simulink model "iff_sim"  (R2019b)
settings: Solver=VariableStepAuto  StartTime=0.0  StopTime=T  FixedStep=0.001  MaxStep=0.01  RelTol=1e-3
values from neighbouring files (symbols this model uses):
  bsc = 17    [model.mat]
  d_r = [0.01 0.01 0.01 0.01 0.01 0.01]    [model.mat]
  Fi_b_z = in_rlb(12,1)    [fcn_s_rlb.m]    (also in fcn_s_rub.m = in_rub(12,1); model.mat = [0 2.09439510239 4.18879020479 1.0471975512 3.14159265359 5.)
  ka = 11860000    [model.mat]
  ksc = 179000    [model.mat]
  l_r = in_rlb(3,1)    [fcn_s_rlb.m]    (also in fcn_s_rub.m = in_rub(3,1); model.mat = [0.36 0.36 0.36 0.36 0.36 0.36])
  la00 = 0.061    [model.mat]
  linderiv = 0    [model.mat]
  O_lb = in_rlb(4:9,1)    [fcn_s_rlb.m]    (also in model.mat = [0 0 0 0 0 0])
  s_0 = s_d(:,:,1)    [iff_run.m]
  t_dist = 0.1    [model.mat]
  ts_noise = 0.00016    [model.mat]
  v_0 = v_d(:,:,1)    [iff_run.m]
  w_lb = in_rlb(11,1)    [fcn_s_rlb.m]    (also in model.mat = 0.195)
  W_lb = 0.205    [model.mat]
  w_ub = in_rub(11,1)    [fcn_s_rub.m]    (also in model.mat = 0.195)
  W_ub = 0.205    [model.mat]
undefined symbols (not defined in the file or in its folder): Kd, Kdiag, Ki, Kp, q_d, qt_d, qtt_d, t_d, X, Y, Z
libraries: nesl_utility x282, sm_lib x208, dspindex x30, simulink_extras x24, simulink x14, powerlib_meascontrol x1
(part 5 of 14)

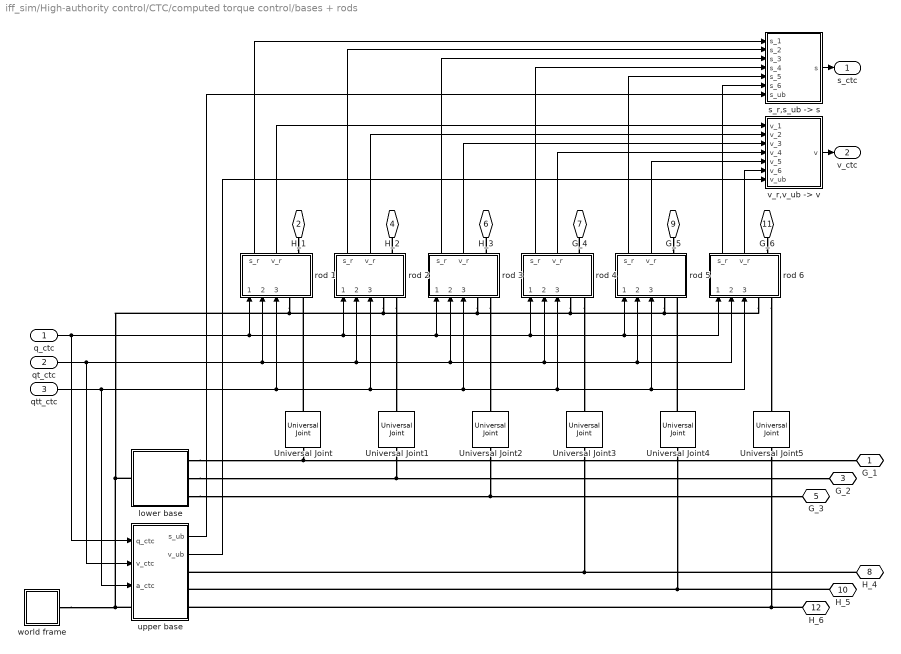
== system iff_sim/High-authority control/CTC/computed torque control/bases + rods ==
  q_ctc : Inport
  qt_ctc : Inport  Port=2
  qtt_ctc : Inport  Port=3
  Universal Joint{,1..5} (6 alike) : sm_lib/Joints/Universal Joint  JointMode=Normal  SenseConstraintForce=off  SenseConstraintForceX=off  SenseConstraintForceY=off  SenseConstraintForceZ=off  SenseConstraintTorque=off  SenseConstraintTorqueX=off  SenseConstraintTorqueY=off  SenseConstraintTorqueZ=off  SenseTotalForce=off  SenseTotalForceX=off  SenseTotalForceY=off  SenseTotalForceZ=off  SenseTotalTorque=off  SenseTotalTorqueX=off  SenseTotalTorqueY=off  SenseTotalTorqueZ=off  CompositeWrenchDir=FollowerOnBase  CompositeWrenchFrame=BaseFrame  RxEquilibriumPosition=0  RxEquilibriumPositionUnits=deg  RxSpringStiffness=0  RxSpringStiffnessUnits=N*m/deg  RxDampingCoefficient=0  RxDampingCoefficientUnits=N*m/(deg/s)  RxTorqueActuationMode=NoTorque  RxMotionActuationMode=ComputedMotion  RxSensePosition=off  RxSenseVelocity=off  RxSenseAcceleration=off  RxSenseTorqueForce=off  RxSenseLowerLimitTorqueForce=off  RxSenseUpperLimitTorqueForce=off  RxLowerLimitSpecify=off  RxLowerLimitBound=-90  RxLowerLimitBoundUnits=deg  RxLowerLimitStiffness=1e4  RxLowerLimitStiffnessUnits=N*m/deg  RxLowerLimitDamping=10  RxLowerLimitDampingUnits=N*m/(deg/s)  RxLowerLimitTransitionRegionWidth=0.1  RxLowerLimitTransitionRegionWidthUnits=deg  RxUpperLimitSpecify=off  RxUpperLimitBound=90  RxUpperLimitBoundUnits=deg  RxUpperLimitStiffness=1e4  RxUpperLimitStiffnessUnits=N*m/deg  RxUpperLimitDamping=10  RxUpperLimitDampingUnits=N*m/(deg/s)  RxUpperLimitTransitionRegionWidth=0.1  RxUpperLimitTransitionRegionWidthUnits=deg  RxPositionTargetSpecify=off  RxPositionTargetPriority=High  RxPositionTargetValue=0  RxPositionTargetValueUnits=deg  RxVelocityTargetSpecify=off  RxVelocityTargetPriority=High  RxVelocityTargetValue=0  RxVelocityTargetValueUnits=deg/s  RyEquilibriumPosition=0  RyEquilibriumPositionUnits=deg  RySpringStiffness=0  RySpringStiffnessUnits=N*m/deg  RyDampingCoefficient=0  RyDampingCoefficientUnits=N*m/(deg/s)  RyTorqueActuationMode=NoTorque  RyMotionActuationMode=ComputedMotion  RySensePosition=off  RySenseVelocity=off  RySenseAcceleration=off  RySenseTorqueForce=off  RySenseLowerLimitTorqueForce=off  RySenseUpperLimitTorqueForce=off  RyLowerLimitSpecify=off  RyLowerLimitBound=-90  RyLowerLimitBoundUnits=deg  RyLowerLimitStiffness=1e4  RyLowerLimitStiffnessUnits=N*m/deg  RyLowerLimitDamping=10  RyLowerLimitDampingUnits=N*m/(deg/s)  RyLowerLimitTransitionRegionWidth=0.1  RyLowerLimitTransitionRegionWidthUnits=deg  RyUpperLimitSpecify=off  RyUpperLimitBound=90  RyUpperLimitBoundUnits=deg  RyUpperLimitStiffness=1e4  RyUpperLimitStiffnessUnits=N*m/deg  RyUpperLimitDamping=10  RyUpperLimitDampingUnits=N*m/(deg/s)  RyUpperLimitTransitionRegionWidth=0.1  RyUpperLimitTransitionRegionWidthUnits=deg  RyPositionTargetSpecify=off  RyPositionTargetPriority=High  RyPositionTargetValue=0  RyPositionTargetValueUnits=deg  RyVelocityTargetSpecify=off  RyVelocityTargetPriority=High  RyVelocityTargetValue=0  RyVelocityTargetValueUnits=deg/s
      settings: SourceProductName=Simscape Multibody
  lower base : Subsystem
  rod 1 : Subsystem  mask{r=1}
  rod 2 : Subsystem  mask{r=2}
  rod 3 : Subsystem  mask{r=3}
  rod 4 : Subsystem  mask{r=4}
  rod 5 : Subsystem  mask{r=5}
  rod 6 : Subsystem  mask{r=6}
  "s_r,s_ub -> s" : MATLAB Function  TreatAsAtomicUnit=on
  upper base : Subsystem
  "v_r,v_ub -> v" : MATLAB Function  TreatAsAtomicUnit=on
  world frame : Subsystem
  G_1 : PMIOPort  Side=Right
  H_1 : PMIOPort  Port=2  Side=Right
  G_2 : PMIOPort  Port=3  Side=Right
  H_2 : PMIOPort  Port=4  Side=Right
  G_3 : PMIOPort  Port=5  Side=Right
  H_3 : PMIOPort  Port=6  Side=Right
  G_4 : PMIOPort  Port=7  Side=Right
  H_4 : PMIOPort  Port=8  Side=Right
  G_5 : PMIOPort  Port=9  Side=Right
  H_5 : PMIOPort  Port=10  Side=Right
  G_6 : PMIOPort  Port=11  Side=Right
  H_6 : PMIOPort  Port=12  Side=Right
  s_ctc : Outport
  v_ctc : Outport  Port=2
  wires:
  q_ctc/1 -> upper base/1(q_ctc), rod 2/1(q_ctc), rod 3/1(q_ctc), rod 4/1(q_ctc), rod 6/1(q_ctc), rod 5/1(q_ctc), rod 1/1(q_ctc)
  qt_ctc/1 -> upper base/2(v_ctc), rod 2/2(v_ctc), rod 3/2(v_ctc), rod 4/2(v_ctc), rod 6/2(v_ctc), rod 5/2(v_ctc), rod 1/2(v_ctc)
  qtt_ctc/1 -> upper base/3(a_ctc), rod 2/3(a_ctc), rod 3/3(a_ctc), rod 4/3(a_ctc), rod 6/3(a_ctc), rod 5/3(a_ctc), rod 1/3(a_ctc)
  rod 4/1(s_r) -> "s_r,s_ub -> s"/4(s_4)
  rod 3/1(s_r) -> "s_r,s_ub -> s"/3(s_3)
  rod 2/1(s_r) -> "s_r,s_ub -> s"/2(s_2)
  rod 1/1(s_r) -> "s_r,s_ub -> s"/1(s_1)
  "s_r,s_ub -> s"/1(s) -> s_ctc/1
  upper base/1(s_ub) -> "s_r,s_ub -> s"/7(s_ub)
  "v_r,v_ub -> v"/1(v) -> v_ctc/1
  rod 4/2(v_r) -> "v_r,v_ub -> v"/4(v_4)
  rod 3/2(v_r) -> "v_r,v_ub -> v"/3(v_3)
  rod 2/2(v_r) -> "v_r,v_ub -> v"/2(v_2)
  rod 1/2(v_r) -> "v_r,v_ub -> v"/1(v_1)
  upper base/2(v_ub) -> "v_r,v_ub -> v"/7(v_ub)
  rod 5/1(s_r) -> "s_r,s_ub -> s"/5(s_5)
  rod 6/1(s_r) -> "s_r,s_ub -> s"/6(s_6)
  rod 5/2(v_r) -> "v_r,v_ub -> v"/5(v_5)
  rod 6/2(v_r) -> "v_r,v_ub -> v"/6(v_6)
  connections:
  lower base/RConn1 -- Universal Joint/LConn1 -- G_1/RConn1
  lower base/RConn2 -- G_2/RConn1 -- Universal Joint1/LConn1
  lower base/RConn3 -- G_3/RConn1 -- Universal Joint2/LConn1
  Universal Joint3/LConn1 -- H_4/RConn1 -- upper base/RConn1
  Universal Joint4/LConn1 -- H_5/RConn1 -- upper base/RConn2
  H_6/RConn1 -- Universal Joint5/LConn1 -- upper base/RConn3
  H_1/RConn1 -- rod 1/RConn1
  Universal Joint/RConn1 -- rod 1/LConn2
  rod 2/LConn2 -- Universal Joint1/RConn1
  rod 2/RConn1 -- H_2/RConn1
  rod 3/RConn1 -- H_3/RConn1
  world frame/RConn1 -- upper base/LConn1 -- lower base/LConn1 -- rod 1/LConn1 -- rod 2/LConn1 -- rod 3/LConn1 -- rod 4/LConn1 -- rod 6/LConn1 -- rod 5/LConn1
  rod 3/LConn2 -- Universal Joint2/RConn1
  rod 4/LConn2 -- Universal Joint3/RConn1
  rod 4/RConn1 -- G_4/RConn1
  Universal Joint4/RConn1 -- rod 5/LConn2
  G_5/RConn1 -- rod 5/RConn1
  G_6/RConn1 -- rod 6/RConn1
  rod 6/LConn2 -- Universal Joint5/RConn1

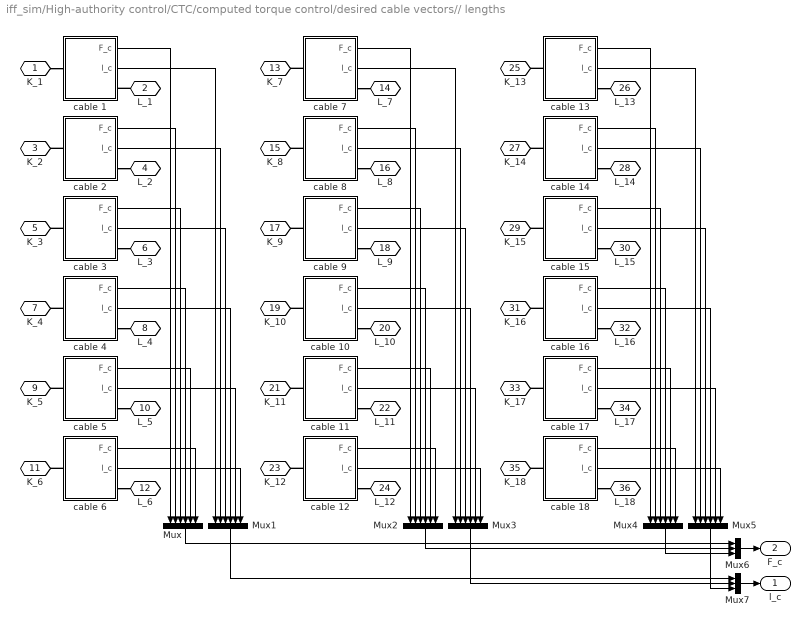
== system iff_sim/High-authority control/CTC/computed torque control/desired cable vectors// lengths ==
  Mux{,1..5} (6 alike) : Mux  Inputs=6
  Mux6 : Mux  Inputs=3
  Mux7 : Mux  Inputs=3
  cable 1 : Subsystem
  cable 10 : Subsystem
  cable 11 : Subsystem
  cable 12 : Subsystem
  cable 13 : Subsystem
  cable 14 : Subsystem
  cable 15 : Subsystem
  cable 16 : Subsystem
  cable 17 : Subsystem
  cable 18 : Subsystem
  cable 2 : Subsystem
  cable 3 : Subsystem
  cable 4 : Subsystem
  cable 5 : Subsystem
  cable 6 : Subsystem
  cable 7 : Subsystem
  cable 8 : Subsystem
  cable 9 : Subsystem
  K_1 : PMIOPort  Side=Left
  L_1 : PMIOPort  Port=2  Side=Left
  K_2 : PMIOPort  Port=3  Side=Left
  L_2 : PMIOPort  Port=4  Side=Left
  K_3 : PMIOPort  Port=5  Side=Left
  L_3 : PMIOPort  Port=6  Side=Left
  K_4 : PMIOPort  Port=7  Side=Left
  L_4 : PMIOPort  Port=8  Side=Left
  K_5 : PMIOPort  Port=9  Side=Left
  L_5 : PMIOPort  Port=10  Side=Left
  K_6 : PMIOPort  Port=11  Side=Left
  L_6 : PMIOPort  Port=12  Side=Left
  K_7 : PMIOPort  Port=13  Side=Left
  L_7 : PMIOPort  Port=14  Side=Left
  K_8 : PMIOPort  Port=15  Side=Left
  L_8 : PMIOPort  Port=16  Side=Left
  K_9 : PMIOPort  Port=17  Side=Left
  L_9 : PMIOPort  Port=18  Side=Left
  K_10 : PMIOPort  Port=19  Side=Left
  L_10 : PMIOPort  Port=20  Side=Left
  K_11 : PMIOPort  Port=21  Side=Left
  L_11 : PMIOPort  Port=22  Side=Left
  K_12 : PMIOPort  Port=23  Side=Left
  L_12 : PMIOPort  Port=24  Side=Left
  K_13 : PMIOPort  Port=25  Side=Left
  L_13 : PMIOPort  Port=26  Side=Left
  K_14 : PMIOPort  Port=27  Side=Left
  L_14 : PMIOPort  Port=28  Side=Left
  K_15 : PMIOPort  Port=29  Side=Left
  L_15 : PMIOPort  Port=30  Side=Left
  K_16 : PMIOPort  Port=31  Side=Left
  L_16 : PMIOPort  Port=32  Side=Left
  K_17 : PMIOPort  Port=33  Side=Left
  L_17 : PMIOPort  Port=34  Side=Left
  K_18 : PMIOPort  Port=35  Side=Left
  L_18 : PMIOPort  Port=36  Side=Left
  l_c : Outport
  F_c : Outport  Port=2
  wires:
  cable 1/1(F_c) -> Mux/1
  cable 2/1(F_c) -> Mux/2
  cable 3/1(F_c) -> Mux/3
  cable 4/1(F_c) -> Mux/4
  cable 5/1(F_c) -> Mux/5
  cable 6/1(F_c) -> Mux/6
  cable 1/2(l_c) -> Mux1/1
  cable 2/2(l_c) -> Mux1/2
  cable 3/2(l_c) -> Mux1/3
  cable 4/2(l_c) -> Mux1/4
  cable 5/2(l_c) -> Mux1/5
  cable 6/2(l_c) -> Mux1/6
  cable 8/2(l_c) -> Mux3/2
  cable 9/1(F_c) -> Mux2/3
  cable 11/1(F_c) -> Mux2/5
  cable 10/2(l_c) -> Mux3/4
  cable 12/2(l_c) -> Mux3/6
  cable 12/1(F_c) -> Mux2/6
  cable 9/2(l_c) -> Mux3/3
  cable 11/2(l_c) -> Mux3/5
  cable 10/1(F_c) -> Mux2/4
  cable 7/1(F_c) -> Mux2/1
  cable 7/2(l_c) -> Mux3/1
  cable 8/1(F_c) -> Mux2/2
  cable 14/2(l_c) -> Mux5/2
  cable 15/1(F_c) -> Mux4/3
  cable 17/1(F_c) -> Mux4/5
  cable 16/2(l_c) -> Mux5/4
  cable 18/2(l_c) -> Mux5/6
  cable 18/1(F_c) -> Mux4/6
  cable 15/2(l_c) -> Mux5/3
  cable 17/2(l_c) -> Mux5/5
  cable 16/1(F_c) -> Mux4/4
  cable 13/1(F_c) -> Mux4/1
  cable 13/2(l_c) -> Mux5/1
  cable 14/1(F_c) -> Mux4/2
  Mux6/1 -> F_c/1
  Mux/1 -> Mux6/1
  Mux2/1 -> Mux6/2
  Mux4/1 -> Mux6/3
  Mux7/1 -> l_c/1
  Mux1/1 -> Mux7/1
  Mux3/1 -> Mux7/2
  Mux5/1 -> Mux7/3
  connections:
  K_1/RConn1 -- cable 1/LConn1
  L_1/RConn1 -- cable 1/RConn1
  cable 2/RConn1 -- L_2/RConn1
  cable 2/LConn1 -- K_2/RConn1
  cable 3/LConn1 -- K_3/RConn1
  cable 3/RConn1 -- L_3/RConn1
  cable 6/RConn1 -- L_6/RConn1
  cable 4/LConn1 -- K_4/RConn1
  cable 5/RConn1 -- L_5/RConn1
  cable 4/RConn1 -- L_4/RConn1
  cable 6/LConn1 -- K_6/RConn1
  cable 5/LConn1 -- K_5/RConn1
  cable 12/RConn1 -- L_12/RConn1
  cable 11/RConn1 -- L_11/RConn1
  cable 7/LConn1 -- K_7/RConn1
  cable 7/RConn1 -- L_7/RConn1
  cable 12/LConn1 -- K_12/RConn1
  cable 8/LConn1 -- K_8/RConn1
  cable 9/RConn1 -- L_9/RConn1
  cable 10/RConn1 -- L_10/RConn1
  cable 10/LConn1 -- K_10/RConn1
  cable 8/RConn1 -- L_8/RConn1
  cable 9/LConn1 -- K_9/RConn1
  cable 11/LConn1 -- K_11/RConn1
  cable 18/RConn1 -- L_18/RConn1
  cable 17/RConn1 -- L_17/RConn1
  cable 13/LConn1 -- K_13/RConn1
  cable 18/LConn1 -- K_18/RConn1
  cable 13/RConn1 -- L_13/RConn1
  cable 16/RConn1 -- L_16/RConn1
  cable 14/LConn1 -- K_14/RConn1
  cable 14/RConn1 -- L_14/RConn1
  cable 16/LConn1 -- K_16/RConn1
  cable 17/LConn1 -- K_17/RConn1
  cable 15/RConn1 -- L_15/RConn1
  cable 15/LConn1 -- K_15/RConn1

== system iff_sim/High-authority control/CTC/computed torque control/q_d,q -> a_ctc ==
  q_d : Inport
  qt_d : Inport  Port=2
  qtt_d : Inport  Port=3
  q : Inport  Port=4
  qt : Inport  Port=5
  Gain : Gain  Gain=Kp
  Gain1 : Gain  Gain=Kd
  Gain2 : Gain  Gain=Ki
  Integrator : Integrator
  Sum : Sum  Inputs=+-|
  Sum1 : Sum  Inputs=+-|
  Sum2 : Sum  Inputs=++++
  To Workspace : ToWorkspace  VariableName=e  SampleTime=-1
  q_ctc : Outport
  qt_ctc : Outport  Port=2
  qtt_ctc : Outport  Port=3
  wires:
  q_d/1 -> Sum/1, q_ctc/1
  qt_d/1 -> Sum1/1, qt_ctc/1
  q/1 -> Sum/2
  qt/1 -> Sum1/2
  Sum2/1 -> qtt_ctc/1
  qtt_d/1 -> Sum2/1
  Sum/1 -> Integrator/1, Gain/1, To Workspace/1
  Gain/1 -> Sum2/2
  Sum1/1 -> Gain1/1
  Gain1/1 -> Sum2/3
  Gain2/1 -> Sum2/4
  Integrator/1 -> Gain2/1

== system iff_sim/High-authority control/CTC/computed torque control/scope q_ctc ==
  in : Inport
  Multiport Selector : dspindex/Multiport Selector  rowsOrCols=Rows  idxCellArray={ 1,2,3,4,5,6}  idxErrMode=Clip Index
  Multiport Selector1 : dspindex/Multiport Selector  rowsOrCols=Rows  idxCellArray={ 7,8,9,10,11,12}  idxErrMode=Clip Index
  Multiport Selector2 : dspindex/Multiport Selector  rowsOrCols=Rows  idxCellArray={ 13,14,15,16,17,18}  idxErrMode=Clip Index
  r = 1-3 : Scope  NumInputPorts=6
  r = 4-6 : Scope  NumInputPorts=6
  ub : Scope  NumInputPorts=6
  wires:
  Multiport Selector/1 -> r = 1-3/1
  Multiport Selector2/2 -> ub/2
  in/1 -> Multiport Selector2/1, Multiport Selector/1, Multiport Selector1/1
  Multiport Selector/2 -> r = 1-3/2
  Multiport Selector1/5 -> r = 4-6/5
  Multiport Selector2/4 -> ub/4
  Multiport Selector/5 -> r = 1-3/5
  Multiport Selector/6 -> r = 1-3/6
  Multiport Selector2/1 -> ub/1
  Multiport Selector/3 -> r = 1-3/3
  Multiport Selector2/5 -> ub/5
  Multiport Selector/4 -> r = 1-3/4
  Multiport Selector1/6 -> r = 4-6/6
  Multiport Selector1/2 -> r = 4-6/2
  Multiport Selector1/4 -> r = 4-6/4
  Multiport Selector1/3 -> r = 4-6/3
  Multiport Selector1/1 -> r = 4-6/1
  Multiport Selector2/3 -> ub/3
  Multiport Selector2/6 -> ub/6

== system iff_sim/High-authority control/CTC/computed torque control/scope qt_ctc ==
  in : Inport
  Multiport Selector : dspindex/Multiport Selector  rowsOrCols=Rows  idxCellArray={ 1,2,3,4,5,6}  idxErrMode=Clip Index
  Multiport Selector1 : dspindex/Multiport Selector  rowsOrCols=Rows  idxCellArray={ 7,8,9,10,11,12}  idxErrMode=Clip Index
  Multiport Selector2 : dspindex/Multiport Selector  rowsOrCols=Rows  idxCellArray={ 13,14,15,16,17,18}  idxErrMode=Clip Index
  r = 1-3 : Scope  NumInputPorts=6
  r = 4-6 : Scope  NumInputPorts=6
  ub : Scope  NumInputPorts=6
  wires:
  Multiport Selector/1 -> r = 1-3/1
  Multiport Selector2/2 -> ub/2
  in/1 -> Multiport Selector2/1, Multiport Selector/1, Multiport Selector1/1
  Multiport Selector/2 -> r = 1-3/2
  Multiport Selector1/5 -> r = 4-6/5
  Multiport Selector2/4 -> ub/4
  Multiport Selector/5 -> r = 1-3/5
  Multiport Selector/6 -> r = 1-3/6
  Multiport Selector2/1 -> ub/1
  Multiport Selector/3 -> r = 1-3/3
  Multiport Selector2/5 -> ub/5
  Multiport Selector/4 -> r = 1-3/4
  Multiport Selector1/6 -> r = 4-6/6
  Multiport Selector1/2 -> r = 4-6/2
  Multiport Selector1/4 -> r = 4-6/4
  Multiport Selector1/3 -> r = 4-6/3
  Multiport Selector1/1 -> r = 4-6/1
  Multiport Selector2/3 -> ub/3
  Multiport Selector2/6 -> ub/6

== system iff_sim/High-authority control/CTC/computed torque control/scope qtt_ctc ==
  in : Inport
  Multiport Selector : dspindex/Multiport Selector  rowsOrCols=Rows  idxCellArray={ 1,2,3,4,5,6}  idxErrMode=Clip Index
  Multiport Selector1 : dspindex/Multiport Selector  rowsOrCols=Rows  idxCellArray={ 7,8,9,10,11,12}  idxErrMode=Clip Index
  Multiport Selector2 : dspindex/Multiport Selector  rowsOrCols=Rows  idxCellArray={ 13,14,15,16,17,18}  idxErrMode=Clip Index
  r = 1-3 : Scope  NumInputPorts=6
  r = 4-6 : Scope  NumInputPorts=6
  ub : Scope  NumInputPorts=6
  wires:
  Multiport Selector/1 -> r = 1-3/1
  Multiport Selector2/2 -> ub/2
  in/1 -> Multiport Selector2/1, Multiport Selector/1, Multiport Selector1/1
  Multiport Selector/2 -> r = 1-3/2
  Multiport Selector1/5 -> r = 4-6/5
  Multiport Selector2/4 -> ub/4
  Multiport Selector/5 -> r = 1-3/5
  Multiport Selector/6 -> r = 1-3/6
  Multiport Selector2/1 -> ub/1
  Multiport Selector/3 -> r = 1-3/3
  Multiport Selector2/5 -> ub/5
  Multiport Selector/4 -> r = 1-3/4
  Multiport Selector1/6 -> r = 4-6/6
  Multiport Selector1/2 -> r = 4-6/2
  Multiport Selector1/4 -> r = 4-6/4
  Multiport Selector1/3 -> r = 4-6/3
  Multiport Selector1/1 -> r = 4-6/1
  Multiport Selector2/3 -> ub/3
  Multiport Selector2/6 -> ub/6

== system iff_sim/High-authority control/CTC/inverse kinematics/t -> q_d ==
  t : Inport
  Mux : Mux  Inputs=7
  rod 1 : Subsystem  mask{r=1}
  rod 2 : Subsystem  mask{r=2}
  rod 3 : Subsystem  mask{r=3}
  rod 4 : Subsystem  mask{r=4}
  rod 5 : Subsystem  mask{r=5}
  rod 6 : Subsystem  mask{r=6}
  upper base : Subsystem
  Q_d : Outport
  wires:
  t/1 -> rod 4/1(t), rod 3/1(t), rod 2/1(t), rod 1/1(t), rod 5/1(t), rod 6/1(t), upper base/1(t)
  rod 2/1(Q_r,d) -> Mux/2
  Mux/1 -> Q_d/1
  rod 4/1(Q_r,d) -> Mux/4
  rod 5/1(Q_r,d) -> Mux/5
  rod 3/1(Q_r,d) -> Mux/3
  rod 1/1(Q_r,d) -> Mux/1
  upper base/1(Q_ub,d) -> Mux/7
  rod 6/1(Q_r,d) -> Mux/6

== system iff_sim/High-authority control/CTC/inverse kinematics/t -> qt_d ==
  t : Inport
  Mux : Mux  Inputs=7
  rod 1 : Subsystem  mask{r=1}
  rod 2 : Subsystem  mask{r=2}
  rod 3 : Subsystem  mask{r=3}
  rod 4 : Subsystem  mask{r=4}
  rod 5 : Subsystem  mask{r=5}
  rod 6 : Subsystem  mask{r=6}
  upper base : Subsystem
  Q_d : Outport
  wires:
  t/1 -> rod 4/1(t), rod 3/1(t), rod 2/1(t), rod 1/1(t), rod 5/1(t), rod 6/1(t), upper base/1(t)
  rod 2/1(Q_r,d) -> Mux/2
  Mux/1 -> Q_d/1
  rod 4/1(Q_r,d) -> Mux/4
  rod 5/1(Q_r,d) -> Mux/5
  rod 3/1(Q_r,d) -> Mux/3
  rod 1/1(Q_r,d) -> Mux/1
  upper base/1(Q_ub,d) -> Mux/7
  rod 6/1(Q_r,d) -> Mux/6

== system iff_sim/High-authority control/CTC/inverse kinematics/t -> qtt_d ==
  t : Inport
  Mux : Mux  Inputs=7
  rod 1 : Subsystem  mask{r=1}
  rod 2 : Subsystem  mask{r=2}
  rod 3 : Subsystem  mask{r=3}
  rod 4 : Subsystem  mask{r=4}
  rod 5 : Subsystem  mask{r=5}
  rod 6 : Subsystem  mask{r=6}
  upper base : Subsystem
  Q_d : Outport
  wires:
  t/1 -> rod 4/1(t), rod 3/1(t), rod 2/1(t), rod 1/1(t), rod 5/1(t), rod 6/1(t), upper base/1(t)
  rod 2/1(Q_r,d) -> Mux/2
  Mux/1 -> Q_d/1
  rod 4/1(Q_r,d) -> Mux/4
  rod 5/1(Q_r,d) -> Mux/5
  rod 3/1(Q_r,d) -> Mux/3
  rod 1/1(Q_r,d) -> Mux/1
  upper base/1(Q_ub,d) -> Mux/7
  rod 6/1(Q_r,d) -> Mux/6

== system iff_sim/dynamic model/Cable dynamics/Real cable forces with spools and piezoactuators/Derivative1 ==
  In1 : Inport  PortDimensions=6
  Constant : Constant
  Derivative : Subsystem  mask{LinOn=linderiv, c=1e4}
      mask prompts: LinOn "Switch value (1 for linearization, 0 for simulation):"; c "Derivative constant  Ns/(s+N):"
  Min : MinMax  Inputs=2
  Product : Product
  Ramp : simulink/Sources/Ramp  slope=1/t_dist  start=0  InitialOutput=0
  Out1 : Outport
  wires:
  Derivative/1(Out1) -> Product/1
  In1/1 -> Derivative/1(In1)
  Product/1 -> Out1/1
  Constant/1 -> Min/2
  Ramp/1 -> Min/1
  Min/1 -> Product/2

== system iff_sim/dynamic model/Cable dynamics/Real cable forces with spools only/Derivative ==
  In1 : Inport  PortDimensions=18
  Constant : Constant
  Derivative : Subsystem  mask{LinOn=linderiv, c=1e4}
      mask prompts: LinOn "Switch value (1 for linearization, 0 for simulation):"; c "Derivative constant  Ns/(s+N):"
  Min : MinMax  Inputs=2
  Product : Product
  Ramp : simulink/Sources/Ramp  slope=1/t_dist  start=0  InitialOutput=0
  Scope : Scope
  Out1 : Outport
  wires:
  Ramp/1 -> Min/1
  Derivative/1(Out1) -> Product/1
  Constant/1 -> Min/2
  In1/1 -> Derivative/1(In1)
  Product/1 -> Scope/1, Out1/1
  Min/1 -> Product/2

== system iff_sim/dynamic model/rods + bases/lower base/O_lb -> G_1 ==
  rot z : sm_lib/Frames and Transforms/Rigid Transform  TranslationMethod=None  TranslationStandardOffset=0  TranslationLengthUnit=m  TranslationStandardAxis=+Z  TranslationCartesianOffset=[0 0 0]  TranslationROffset=0  TranslationROffsetUnits=m  TranslationZOffset=0  TranslationZOffsetUnits=m  TranslationThetaOffset=0  TranslationThetaOffsetUnits=deg  RotationMethod=StandardAxis  RotationAngleUnits=rad  RotationStandardAxis=+Z  RotationAngle=Fi_b_z(1)  RotationArbitraryAxis=[0 0 1]  FollAlignAxisA=+X  BaseAlignAxisA=+Y  FollAlignAxisB=+Y  BaseAlignAxisB=+Z  RotationSequenceAxes=FollowerAxes  RotationSequence=XYX  RotationSequenceAngles=[0 0 0]  RotationSequenceAnglesUnits=deg  RotationMatrix=[1 0 0; 0 1 0; 0 0 1]
  trans z : sm_lib/Frames and Transforms/Rigid Transform  TranslationMethod=StandardAxis  TranslationStandardOffset=h_lb  TranslationLengthUnit=m  TranslationStandardAxis=+Z  TranslationCartesianOffset=[0 0 0]  TranslationROffset=0  TranslationROffsetUnits=m  TranslationZOffset=0  TranslationZOffsetUnits=m  TranslationThetaOffset=0  TranslationThetaOffsetUnits=deg  RotationMethod=None  RotationAngleUnits=deg  RotationStandardAxis=+Z  RotationAngle=0.0  RotationArbitraryAxis=[0 0 1]  FollAlignAxisA=+X  BaseAlignAxisA=+Y  FollAlignAxisB=+Y  BaseAlignAxisB=+Z  RotationSequenceAxes=FollowerAxes  RotationSequence=XYX  RotationSequenceAngles=[0 0 0]  RotationSequenceAnglesUnits=deg  RotationMatrix=[1 0 0; 0 1 0; 0 0 1]
  transl y : sm_lib/Frames and Transforms/Rigid Transform  TranslationMethod=StandardAxis  TranslationStandardOffset=w_lb/2  TranslationLengthUnit=m  TranslationStandardAxis=+Y  TranslationCartesianOffset=[0 0 0]  TranslationROffset=0  TranslationROffsetUnits=m  TranslationZOffset=0  TranslationZOffsetUnits=m  TranslationThetaOffset=0  TranslationThetaOffsetUnits=deg  RotationMethod=None  RotationAngleUnits=deg  RotationStandardAxis=+Z  RotationAngle=0.0  RotationArbitraryAxis=[0 0 1]  FollAlignAxisA=+X  BaseAlignAxisA=+Y  FollAlignAxisB=+Y  BaseAlignAxisB=+Z  RotationSequenceAxes=FollowerAxes  RotationSequence=XYX  RotationSequenceAngles=[0 0 0]  RotationSequenceAnglesUnits=deg  RotationMatrix=[1 0 0; 0 1 0; 0 0 1]
  O_lb : PMIOPort  Side=Left
  G_1 : PMIOPort  Port=2  Side=Right
  connections:
  trans z/LConn1 -- O_lb/RConn1
  trans z/RConn1 -- rot z/LConn1
  transl y/LConn1 -- rot z/RConn1
  transl y/RConn1 -- G_1/RConn1

== system iff_sim/dynamic model/rods + bases/lower base/O_lb -> G_2 ==
  rot z : sm_lib/Frames and Transforms/Rigid Transform  TranslationMethod=None  TranslationStandardOffset=0  TranslationLengthUnit=m  TranslationStandardAxis=+Z  TranslationCartesianOffset=[0 0 0]  TranslationROffset=0  TranslationROffsetUnits=m  TranslationZOffset=0  TranslationZOffsetUnits=m  TranslationThetaOffset=0  TranslationThetaOffsetUnits=deg  RotationMethod=StandardAxis  RotationAngleUnits=rad  RotationStandardAxis=+Z  RotationAngle=Fi_b_z(2)  RotationArbitraryAxis=[0 0 1]  FollAlignAxisA=+X  BaseAlignAxisA=+Y  FollAlignAxisB=+Y  BaseAlignAxisB=+Z  RotationSequenceAxes=FollowerAxes  RotationSequence=XYX  RotationSequenceAngles=[0 0 0]  RotationSequenceAnglesUnits=deg  RotationMatrix=[1 0 0; 0 1 0; 0 0 1]
  trans z : sm_lib/Frames and Transforms/Rigid Transform  TranslationMethod=StandardAxis  TranslationStandardOffset=h_lb  TranslationLengthUnit=m  TranslationStandardAxis=+Z  TranslationCartesianOffset=[0 0 0]  TranslationROffset=0  TranslationROffsetUnits=m  TranslationZOffset=0  TranslationZOffsetUnits=m  TranslationThetaOffset=0  TranslationThetaOffsetUnits=deg  RotationMethod=None  RotationAngleUnits=deg  RotationStandardAxis=+Z  RotationAngle=0.0  RotationArbitraryAxis=[0 0 1]  FollAlignAxisA=+X  BaseAlignAxisA=+Y  FollAlignAxisB=+Y  BaseAlignAxisB=+Z  RotationSequenceAxes=FollowerAxes  RotationSequence=XYX  RotationSequenceAngles=[0 0 0]  RotationSequenceAnglesUnits=deg  RotationMatrix=[1 0 0; 0 1 0; 0 0 1]
  transl y : sm_lib/Frames and Transforms/Rigid Transform  TranslationMethod=StandardAxis  TranslationStandardOffset=w_lb/2  TranslationLengthUnit=m  TranslationStandardAxis=+Y  TranslationCartesianOffset=[0 0 0]  TranslationROffset=0  TranslationROffsetUnits=m  TranslationZOffset=0  TranslationZOffsetUnits=m  TranslationThetaOffset=0  TranslationThetaOffsetUnits=deg  RotationMethod=None  RotationAngleUnits=deg  RotationStandardAxis=+Z  RotationAngle=0.0  RotationArbitraryAxis=[0 0 1]  FollAlignAxisA=+X  BaseAlignAxisA=+Y  FollAlignAxisB=+Y  BaseAlignAxisB=+Z  RotationSequenceAxes=FollowerAxes  RotationSequence=XYX  RotationSequenceAngles=[0 0 0]  RotationSequenceAnglesUnits=deg  RotationMatrix=[1 0 0; 0 1 0; 0 0 1]
  O_lb : PMIOPort  Side=Left
  G_1 : PMIOPort  Port=2  Side=Right
  connections:
  trans z/LConn1 -- O_lb/RConn1
  trans z/RConn1 -- rot z/LConn1
  transl y/LConn1 -- rot z/RConn1
  transl y/RConn1 -- G_1/RConn1

== system iff_sim/dynamic model/rods + bases/lower base/O_lb -> G_3 ==
  rot z : sm_lib/Frames and Transforms/Rigid Transform  TranslationMethod=None  TranslationStandardOffset=0  TranslationLengthUnit=m  TranslationStandardAxis=+Z  TranslationCartesianOffset=[0 0 0]  TranslationROffset=0  TranslationROffsetUnits=m  TranslationZOffset=0  TranslationZOffsetUnits=m  TranslationThetaOffset=0  TranslationThetaOffsetUnits=deg  RotationMethod=StandardAxis  RotationAngleUnits=rad  RotationStandardAxis=+Z  RotationAngle=Fi_b_z(3)  RotationArbitraryAxis=[0 0 1]  FollAlignAxisA=+X  BaseAlignAxisA=+Y  FollAlignAxisB=+Y  BaseAlignAxisB=+Z  RotationSequenceAxes=FollowerAxes  RotationSequence=XYX  RotationSequenceAngles=[0 0 0]  RotationSequenceAnglesUnits=deg  RotationMatrix=[1 0 0; 0 1 0; 0 0 1]
  trans z : sm_lib/Frames and Transforms/Rigid Transform  TranslationMethod=StandardAxis  TranslationStandardOffset=h_lb  TranslationLengthUnit=m  TranslationStandardAxis=+Z  TranslationCartesianOffset=[0 0 0]  TranslationROffset=0  TranslationROffsetUnits=m  TranslationZOffset=0  TranslationZOffsetUnits=m  TranslationThetaOffset=0  TranslationThetaOffsetUnits=deg  RotationMethod=None  RotationAngleUnits=deg  RotationStandardAxis=+Z  RotationAngle=0.0  RotationArbitraryAxis=[0 0 1]  FollAlignAxisA=+X  BaseAlignAxisA=+Y  FollAlignAxisB=+Y  BaseAlignAxisB=+Z  RotationSequenceAxes=FollowerAxes  RotationSequence=XYX  RotationSequenceAngles=[0 0 0]  RotationSequenceAnglesUnits=deg  RotationMatrix=[1 0 0; 0 1 0; 0 0 1]
  transl y : sm_lib/Frames and Transforms/Rigid Transform  TranslationMethod=StandardAxis  TranslationStandardOffset=w_lb/2  TranslationLengthUnit=m  TranslationStandardAxis=+Y  TranslationCartesianOffset=[0 0 0]  TranslationROffset=0  TranslationROffsetUnits=m  TranslationZOffset=0  TranslationZOffsetUnits=m  TranslationThetaOffset=0  TranslationThetaOffsetUnits=deg  RotationMethod=None  RotationAngleUnits=deg  RotationStandardAxis=+Z  RotationAngle=0.0  RotationArbitraryAxis=[0 0 1]  FollAlignAxisA=+X  BaseAlignAxisA=+Y  FollAlignAxisB=+Y  BaseAlignAxisB=+Z  RotationSequenceAxes=FollowerAxes  RotationSequence=XYX  RotationSequenceAngles=[0 0 0]  RotationSequenceAnglesUnits=deg  RotationMatrix=[1 0 0; 0 1 0; 0 0 1]
  O_lb : PMIOPort  Side=Left
  G_1 : PMIOPort  Port=2  Side=Right
  connections:
  trans z/LConn1 -- O_lb/RConn1
  trans z/RConn1 -- rot z/LConn1
  transl y/LConn1 -- rot z/RConn1
  transl y/RConn1 -- G_1/RConn1

== system iff_sim/dynamic model/rods + bases/lower base/wf -> O_lb ==
  vib : Inport
  Bushing Joint : sm_lib/Joints/Bushing Joint  JointMode=Normal  SenseConstraintForce=off  SenseConstraintForceX=off  SenseConstraintForceY=off  SenseConstraintForceZ=off  SenseConstraintTorque=off  SenseConstraintTorqueX=off  SenseConstraintTorqueY=off  SenseConstraintTorqueZ=off  SenseTotalForce=off  SenseTotalForceX=off  SenseTotalForceY=off  SenseTotalForceZ=off  SenseTotalTorque=off  SenseTotalTorqueX=off  SenseTotalTorqueY=off  SenseTotalTorqueZ=off  CompositeWrenchDir=FollowerOnBase  CompositeWrenchFrame=BaseFrame  PxEquilibriumPosition=0  PxEquilibriumPositionUnits=m  PxSpringStiffness=0  PxSpringStiffnessUnits=N/m  PxDampingCoefficient=0  PxDampingCoefficientUnits=N/(m/s)  PxTorqueActuationMode=ComputedTorque  PxMotionActuationMode=InputMotion  PxSensePosition=off  PxSenseVelocity=off  PxSenseAcceleration=off  PxSenseTorqueForce=off  PxSenseLowerLimitTorqueForce=off  PxSenseUpperLimitTorqueForce=off  PxLowerLimitSpecify=off  PxLowerLimitBound=-1  PxLowerLimitBoundUnits=m  PxLowerLimitStiffness=1e6  PxLowerLimitStiffnessUnits=N/m  PxLowerLimitDamping=1e3  PxLowerLimitDampingUnits=N/(m/s)  PxLowerLimitTransitionRegionWidth=1e-4  PxLowerLimitTransitionRegionWidthUnits=m  PxUpperLimitSpecify=off  PxUpperLimitBound=1  PxUpperLimitBoundUnits=m  PxUpperLimitStiffness=1e6  PxUpperLimitStiffnessUnits=N/m  PxUpperLimitDamping=1e3  PxUpperLimitDampingUnits=N/(m/s)  PxUpperLimitTransitionRegionWidth=1e-4  PxUpperLimitTransitionRegionWidthUnits=m  PxPositionTargetSpecify=off  PxPositionTargetPriority=High  PxPositionTargetValue=0  PxPositionTargetValueUnits=m  PxVelocityTargetSpecify=off  PxVelocityTargetPriority=High  PxVelocityTargetValue=0  PxVelocityTargetValueUnits=m/s  PyEquilibriumPosition=0  PyEquilibriumPositionUnits=m  PySpringStiffness=0  PySpringStiffnessUnits=N/m  PyDampingCoefficient=0  PyDampingCoefficientUnits=N/(m/s)  PyTorqueActuationMode=ComputedTorque  PyMotionActuationMode=InputMotion  PySensePosition=off  PySenseVelocity=off  PySenseAcceleration=off  PySenseTorqueForce=off  PySenseLowerLimitTorqueForce=off  PySenseUpperLimitTorqueForce=off  PyLowerLimitSpecify=off  PyLowerLimitBound=-1  PyLowerLimitBoundUnits=m  PyLowerLimitStiffness=1e6  PyLowerLimitStiffnessUnits=N/m  PyLowerLimitDamping=1e3  PyLowerLimitDampingUnits=N/(m/s)  PyLowerLimitTransitionRegionWidth=1e-4  PyLowerLimitTransitionRegionWidthUnits=m  PyUpperLimitSpecify=off  PyUpperLimitBound=1  PyUpperLimitBoundUnits=m  PyUpperLimitStiffness=1e6  PyUpperLimitStiffnessUnits=N/m  PyUpperLimitDamping=1e3  PyUpperLimitDampingUnits=N/(m/s)  PyUpperLimitTransitionRegionWidth=1e-4  PyUpperLimitTransitionRegionWidthUnits=m  PyPositionTargetSpecify=off  PyPositionTargetPriority=High  PyPositionTargetValue=0  PyPositionTargetValueUnits=m  PyVelocityTargetSpecify=off  PyVelocityTargetPriority=High  PyVelocityTargetValue=0  PyVelocityTargetValueUnits=m/s  PzEquilibriumPosition=0  PzEquilibriumPositionUnits=m  PzSpringStiffness=0  PzSpringStiffnessUnits=N/m  PzDampingCoefficient=0  PzDampingCoefficientUnits=N/(m/s)  PzTorqueActuationMode=ComputedTorque  PzMotionActuationMode=InputMotion  PzSensePosition=off  PzSenseVelocity=off  PzSenseAcceleration=off  PzSenseTorqueForce=off  PzSenseLowerLimitTorqueForce=off  PzSenseUpperLimitTorqueForce=off  PzLowerLimitSpecify=off  PzLowerLimitBound=-1  PzLowerLimitBoundUnits=m  PzLowerLimitStiffness=1e6  PzLowerLimitStiffnessUnits=N/m  PzLowerLimitDamping=1e3  PzLowerLimitDampingUnits=N/(m/s)  PzLowerLimitTransitionRegionWidth=1e-4  PzLowerLimitTransitionRegionWidthUnits=m  PzUpperLimitSpecify=off  PzUpperLimitBound=1  PzUpperLimitBoundUnits=m  PzUpperLimitStiffness=1e6  PzUpperLimitStiffnessUnits=N/m  PzUpperLimitDamping=1e3  PzUpperLimitDampingUnits=N/(m/s)  PzUpperLimitTransitionRegionWidth=1e-4  PzUpperLimitTransitionRegionWidthUnits=m  PzPositionTargetSpecify=off  PzPositionTargetPriority=High  PzPositionTargetValue=0  PzPositionTargetValueUnits=m  PzVelocityTargetSpecify=off  PzVelocityTargetPriority=High  PzVelocityTargetValue=0  PzVelocityTargetValueUnits=m/s  RxEquilibriumPosition=0  RxEquilibriumPositionUnits=deg  RxSpringStiffness=0  RxSpringStiffnessUnits=N*m/deg  RxDampingCoefficient=0  RxDampingCoefficientUnits=N*m/(deg/s)  RxTorqueActuationMode=ComputedTorque  RxMotionActuationMode=InputMotion  RxSensePosition=off  RxSenseVelocity=off  RxSenseAcceleration=off  RxSenseTorqueForce=off  RxSenseLowerLimitTorqueForce=off  RxSenseUpperLimitTorqueForce=off  RxLowerLimitSpecify=off  RxLowerLimitBound=-90  RxLowerLimitBoundUnits=deg  RxLowerLimitStiffness=1e4  RxLowerLimitStiffnessUnits=N*m/deg  RxLowerLimitDamping=10  RxLowerLimitDampingUnits=N*m/(deg/s)  RxLowerLimitTransitionRegionWidth=0.1  RxLowerLimitTransitionRegionWidthUnits=deg  RxUpperLimitSpecify=off  RxUpperLimitBound=90  RxUpperLimitBoundUnits=deg  RxUpperLimitStiffness=1e4  RxUpperLimitStiffnessUnits=N*m/deg  RxUpperLimitDamping=10  RxUpperLimitDampingUnits=N*m/(deg/s)  RxUpperLimitTransitionRegionWidth=0.1  RxUpperLimitTransitionRegionWidthUnits=deg  RxPositionTargetSpecify=off  RxPositionTargetPriority=High  RxPositionTargetValue=0  RxPositionTargetValueUnits=deg  RxVelocityTargetSpecify=off  RxVelocityTargetPriority=High  RxVelocityTargetValue=0  RxVelocityTargetValueUnits=deg/s  RyEquilibriumPosition=0  RyEquilibriumPositionUnits=deg  RySpringStiffness=0  RySpringStiffnessUnits=N*m/deg  RyDampingCoefficient=0  RyDampingCoefficientUnits=N*m/(deg/s)  RyTorqueActuationMode=ComputedTorque  RyMotionActuationMode=InputMotion  RySensePosition=off  RySenseVelocity=off  RySenseAcceleration=off  RySenseTorqueForce=off  RySenseLowerLimitTorqueForce=off  RySenseUpperLimitTorqueForce=off  RyLowerLimitSpecify=off  RyLowerLimitBound=-90  RyLowerLimitBoundUnits=deg  RyLowerLimitStiffness=1e4  RyLowerLimitStiffnessUnits=N*m/deg  RyLowerLimitDamping=10  RyLowerLimitDampingUnits=N*m/(deg/s)  RyLowerLimitTransitionRegionWidth=0.1  RyLowerLimitTransitionRegionWidthUnits=deg  RyUpperLimitSpecify=off  RyUpperLimitBound=90  RyUpperLimitBoundUnits=deg  RyUpperLimitStiffness=1e4  RyUpperLimitStiffnessUnits=N*m/deg  RyUpperLimitDamping=10  RyUpperLimitDampingUnits=N*m/(deg/s)  RyUpperLimitTransitionRegionWidth=0.1  RyUpperLimitTransitionRegionWidthUnits=deg  RyPositionTargetSpecify=off  RyPositionTargetPriority=High  RyPositionTargetValue=0  RyPositionTargetValueUnits=deg  RyVelocityTargetSpecify=off  RyVelocityTargetPriority=High  RyVelocityTargetValue=0  RyVelocityTargetValueUnits=deg/s  RzEquilibriumPosition=0  RzEquilibriumPositionUnits=deg  RzSpringStiffness=0  RzSpringStiffnessUnits=N*m/deg  RzDampingCoefficient=0  RzDampingCoefficientUnits=N*m/(deg/s)  RzTorqueActuationMode=ComputedTorque  RzMotionActuationMode=InputMotion  RzSensePosition=off  RzSenseVelocity=off  RzSenseAcceleration=off  RzSenseTorqueForce=off  RzSenseLowerLimitTorqueForce=off  RzSenseUpperLimitTorqueForce=off  RzLowerLimitSpecify=off  RzLowerLimitBound=-90  RzLowerLimitBoundUnits=deg  RzLowerLimitStiffness=1e4  RzLowerLimitStiffnessUnits=N*m/deg  RzLowerLimitDamping=10  RzLowerLimitDampingUnits=N*m/(deg/s)  RzLowerLimitTransitionRegionWidth=0.1  RzLowerLimitTransitionRegionWidthUnits=deg  RzUpperLimitSpecify=off  RzUpperLimitBound=90  RzUpperLimitBoundUnits=deg  RzUpperLimitStiffness=1e4  RzUpperLimitStiffnessUnits=N*m/deg  RzUpperLimitDamping=10  RzUpperLimitDampingUnits=N*m/(deg/s)  RzUpperLimitTransitionRegionWidth=0.1  RzUpperLimitTransitionRegionWidthUnits=deg  RzPositionTargetSpecify=off  RzPositionTargetPriority=High  RzPositionTargetValue=0  RzPositionTargetValueUnits=deg  RzVelocityTargetSpecify=off  RzVelocityTargetPriority=High  RzVelocityTargetValue=0  RzVelocityTargetValueUnits=deg/s
      settings: SourceProductName=Simscape Multibody
  Demux : Demux  Outputs=6
  Simulink-PS Converter{,1..5} (6 alike) : nesl_utility/Simulink-PS Converter  PhysicalDomain=network_engine_domain  SubClassName=ps_input  LeftPortType=input  RightPortType=output  PseudoPeriodic=off  Frequencies=[]  NoiseDistribution=none  NoiseParameters=[]  Unit=1  AffineConversion=off  FilteringAndDerivatives=filter  SimscapeFilterOrder=2  InputFilterTimeConstant=0.001  UdotUserProvided=0
  rot x : sm_lib/Frames and Transforms/Rigid Transform  TranslationMethod=None  TranslationStandardOffset=0  TranslationLengthUnit=m  TranslationStandardAxis=+Z  TranslationCartesianOffset=[0 0 0]  TranslationROffset=0  TranslationROffsetUnits=m  TranslationZOffset=0  TranslationZOffsetUnits=m  TranslationThetaOffset=0  TranslationThetaOffsetUnits=deg  RotationMethod=StandardAxis  RotationAngleUnits=rad  RotationStandardAxis=+X  RotationAngle=O_lb(4,1)  RotationArbitraryAxis=[0 0 1]  FollAlignAxisA=+X  BaseAlignAxisA=+Y  FollAlignAxisB=+Y  BaseAlignAxisB=+Z  RotationSequenceAxes=FollowerAxes  RotationSequence=XYX  RotationSequenceAngles=[0 0 0]  RotationSequenceAnglesUnits=deg  RotationMatrix=[1 0 0; 0 1 0; 0 0 1]
  rot y : sm_lib/Frames and Transforms/Rigid Transform  TranslationMethod=None  TranslationStandardOffset=0  TranslationLengthUnit=m  TranslationStandardAxis=+Z  TranslationCartesianOffset=[0 0 0]  TranslationROffset=0  TranslationROffsetUnits=m  TranslationZOffset=0  TranslationZOffsetUnits=m  TranslationThetaOffset=0  TranslationThetaOffsetUnits=deg  RotationMethod=StandardAxis  RotationAngleUnits=rad  RotationStandardAxis=+Y  RotationAngle=O_lb(5,1)  RotationArbitraryAxis=[0 0 1]  FollAlignAxisA=+X  BaseAlignAxisA=+Y  FollAlignAxisB=+Y  BaseAlignAxisB=+Z  RotationSequenceAxes=FollowerAxes  RotationSequence=XYX  RotationSequenceAngles=[0 0 0]  RotationSequenceAnglesUnits=deg  RotationMatrix=[1 0 0; 0 1 0; 0 0 1]
  rot z : sm_lib/Frames and Transforms/Rigid Transform  TranslationMethod=None  TranslationStandardOffset=0  TranslationLengthUnit=m  TranslationStandardAxis=+Z  TranslationCartesianOffset=[0 0 0]  TranslationROffset=0  TranslationROffsetUnits=m  TranslationZOffset=0  TranslationZOffsetUnits=m  TranslationThetaOffset=0  TranslationThetaOffsetUnits=deg  RotationMethod=StandardAxis  RotationAngleUnits=rad  RotationStandardAxis=+X  RotationAngle=O_lb(6,1)  RotationArbitraryAxis=[0 0 1]  FollAlignAxisA=+X  BaseAlignAxisA=+Y  FollAlignAxisB=+Y  BaseAlignAxisB=+Z  RotationSequenceAxes=FollowerAxes  RotationSequence=XYX  RotationSequenceAngles=[0 0 0]  RotationSequenceAnglesUnits=deg  RotationMatrix=[1 0 0; 0 1 0; 0 0 1]
  transl : sm_lib/Frames and Transforms/Rigid Transform  TranslationMethod=Cartesian  TranslationStandardOffset=0  TranslationLengthUnit=m  TranslationStandardAxis=+Z  TranslationCartesianOffset=O_lb(1:3,1)  TranslationROffset=0  TranslationROffsetUnits=m  TranslationZOffset=0  TranslationZOffsetUnits=m  TranslationThetaOffset=0  TranslationThetaOffsetUnits=deg  RotationMethod=None  RotationAngleUnits=deg  RotationStandardAxis=+Z  RotationAngle=0.0  RotationArbitraryAxis=[0 0 1]  FollAlignAxisA=+X  BaseAlignAxisA=+Y  FollAlignAxisB=+Y  BaseAlignAxisB=+Z  RotationSequenceAxes=FollowerAxes  RotationSequence=XYX  RotationSequenceAngles=[0 0 0]  RotationSequenceAnglesUnits=deg  RotationMatrix=[1 0 0; 0 1 0; 0 0 1]
  wf : PMIOPort  Side=Left
  O_lb : PMIOPort  Port=2  Side=Right
  wires:
  Demux/4 -> Simulink-PS Converter3/1
  vib/1 -> Demux/1
  Demux/2 -> Simulink-PS Converter1/1
  Demux/5 -> Simulink-PS Converter4/1
  Demux/1 -> Simulink-PS Converter/1
  Demux/6 -> Simulink-PS Converter5/1
  Demux/3 -> Simulink-PS Converter2/1
  connections:
  transl/RConn1 -- rot x/LConn1
  rot x/RConn1 -- rot y/LConn1
  rot y/RConn1 -- rot z/LConn1
  O_lb/RConn1 -- rot z/RConn1
  Bushing Joint/LConn6 -- Simulink-PS Converter4/RConn1
  Bushing Joint/LConn3 -- Simulink-PS Converter1/RConn1
  Bushing Joint/LConn5 -- Simulink-PS Converter3/RConn1
  Bushing Joint/LConn7 -- Simulink-PS Converter5/RConn1
  Bushing Joint/LConn2 -- Simulink-PS Converter/RConn1
  Bushing Joint/LConn4 -- Simulink-PS Converter2/RConn1
  wf/RConn1 -- Bushing Joint/LConn1
  Bushing Joint/RConn1 -- transl/LConn1

== system iff_sim/dynamic model/rods + bases/upper base/O_ub -> H_4 ==
  rot z : sm_lib/Frames and Transforms/Rigid Transform  TranslationMethod=None  TranslationStandardOffset=0  TranslationLengthUnit=m  TranslationStandardAxis=+Z  TranslationCartesianOffset=[0 0 0]  TranslationROffset=0  TranslationROffsetUnits=m  TranslationZOffset=0  TranslationZOffsetUnits=m  TranslationThetaOffset=0  TranslationThetaOffsetUnits=deg  RotationMethod=StandardAxis  RotationAngleUnits=rad  RotationStandardAxis=+Z  RotationAngle=Fi_b_z(4)  RotationArbitraryAxis=[0 0 1]  FollAlignAxisA=+X  BaseAlignAxisA=+Y  FollAlignAxisB=+Y  BaseAlignAxisB=+Z  RotationSequenceAxes=FollowerAxes  RotationSequence=XYX  RotationSequenceAngles=[0 0 0]  RotationSequenceAnglesUnits=deg  RotationMatrix=[1 0 0; 0 1 0; 0 0 1]
  trans z : sm_lib/Frames and Transforms/Rigid Transform  TranslationMethod=StandardAxis  TranslationStandardOffset=h_ub  TranslationLengthUnit=m  TranslationStandardAxis=-Z  TranslationCartesianOffset=[0 0 0]  TranslationROffset=0  TranslationROffsetUnits=m  TranslationZOffset=0  TranslationZOffsetUnits=m  TranslationThetaOffset=0  TranslationThetaOffsetUnits=deg  RotationMethod=None  RotationAngleUnits=deg  RotationStandardAxis=+Z  RotationAngle=0.0  RotationArbitraryAxis=[0 0 1]  FollAlignAxisA=+X  BaseAlignAxisA=+Y  FollAlignAxisB=+Y  BaseAlignAxisB=+Z  RotationSequenceAxes=FollowerAxes  RotationSequence=XYX  RotationSequenceAngles=[0 0 0]  RotationSequenceAnglesUnits=deg  RotationMatrix=[1 0 0; 0 1 0; 0 0 1]
  transl y : sm_lib/Frames and Transforms/Rigid Transform  TranslationMethod=StandardAxis  TranslationStandardOffset=w_ub/2  TranslationLengthUnit=m  TranslationStandardAxis=+Y  TranslationCartesianOffset=[0 0 0]  TranslationROffset=0  TranslationROffsetUnits=m  TranslationZOffset=0  TranslationZOffsetUnits=m  TranslationThetaOffset=0  TranslationThetaOffsetUnits=deg  RotationMethod=None  RotationAngleUnits=deg  RotationStandardAxis=+Z  RotationAngle=0.0  RotationArbitraryAxis=[0 0 1]  FollAlignAxisA=+X  BaseAlignAxisA=+Y  FollAlignAxisB=+Y  BaseAlignAxisB=+Z  RotationSequenceAxes=FollowerAxes  RotationSequence=XYX  RotationSequenceAngles=[0 0 0]  RotationSequenceAnglesUnits=deg  RotationMatrix=[1 0 0; 0 1 0; 0 0 1]
  O_ub : PMIOPort  Side=Left
  H_4 : PMIOPort  Port=2  Side=Right
  connections:
  trans z/LConn1 -- O_ub/RConn1
  trans z/RConn1 -- rot z/LConn1
  transl y/LConn1 -- rot z/RConn1
  transl y/RConn1 -- H_4/RConn1

== system iff_sim/dynamic model/rods + bases/upper base/O_ub -> H_5 ==
  rot z : sm_lib/Frames and Transforms/Rigid Transform  TranslationMethod=None  TranslationStandardOffset=0  TranslationLengthUnit=m  TranslationStandardAxis=+Z  TranslationCartesianOffset=[0 0 0]  TranslationROffset=0  TranslationROffsetUnits=m  TranslationZOffset=0  TranslationZOffsetUnits=m  TranslationThetaOffset=0  TranslationThetaOffsetUnits=deg  RotationMethod=StandardAxis  RotationAngleUnits=rad  RotationStandardAxis=+Z  RotationAngle=Fi_b_z(5)  RotationArbitraryAxis=[0 0 1]  FollAlignAxisA=+X  BaseAlignAxisA=+Y  FollAlignAxisB=+Y  BaseAlignAxisB=+Z  RotationSequenceAxes=FollowerAxes  RotationSequence=XYX  RotationSequenceAngles=[0 0 0]  RotationSequenceAnglesUnits=deg  RotationMatrix=[1 0 0; 0 1 0; 0 0 1]
  trans z : sm_lib/Frames and Transforms/Rigid Transform  TranslationMethod=StandardAxis  TranslationStandardOffset=h_ub  TranslationLengthUnit=m  TranslationStandardAxis=-Z  TranslationCartesianOffset=[0 0 0]  TranslationROffset=0  TranslationROffsetUnits=m  TranslationZOffset=0  TranslationZOffsetUnits=m  TranslationThetaOffset=0  TranslationThetaOffsetUnits=deg  RotationMethod=None  RotationAngleUnits=deg  RotationStandardAxis=+Z  RotationAngle=0.0  RotationArbitraryAxis=[0 0 1]  FollAlignAxisA=+X  BaseAlignAxisA=+Y  FollAlignAxisB=+Y  BaseAlignAxisB=+Z  RotationSequenceAxes=FollowerAxes  RotationSequence=XYX  RotationSequenceAngles=[0 0 0]  RotationSequenceAnglesUnits=deg  RotationMatrix=[1 0 0; 0 1 0; 0 0 1]
  transl y : sm_lib/Frames and Transforms/Rigid Transform  TranslationMethod=StandardAxis  TranslationStandardOffset=w_ub/2  TranslationLengthUnit=m  TranslationStandardAxis=+Y  TranslationCartesianOffset=[0 0 0]  TranslationROffset=0  TranslationROffsetUnits=m  TranslationZOffset=0  TranslationZOffsetUnits=m  TranslationThetaOffset=0  TranslationThetaOffsetUnits=deg  RotationMethod=None  RotationAngleUnits=deg  RotationStandardAxis=+Z  RotationAngle=0.0  RotationArbitraryAxis=[0 0 1]  FollAlignAxisA=+X  BaseAlignAxisA=+Y  FollAlignAxisB=+Y  BaseAlignAxisB=+Z  RotationSequenceAxes=FollowerAxes  RotationSequence=XYX  RotationSequenceAngles=[0 0 0]  RotationSequenceAnglesUnits=deg  RotationMatrix=[1 0 0; 0 1 0; 0 0 1]
  O_ub : PMIOPort  Side=Left
  H_5 : PMIOPort  Port=2  Side=Right
  connections:
  trans z/LConn1 -- O_ub/RConn1
  trans z/RConn1 -- rot z/LConn1
  transl y/LConn1 -- rot z/RConn1
  transl y/RConn1 -- H_5/RConn1

== system iff_sim/dynamic model/rods + bases/upper base/O_ub -> H_6 ==
  rot z : sm_lib/Frames and Transforms/Rigid Transform  TranslationMethod=None  TranslationStandardOffset=0  TranslationLengthUnit=m  TranslationStandardAxis=+Z  TranslationCartesianOffset=[0 0 0]  TranslationROffset=0  TranslationROffsetUnits=m  TranslationZOffset=0  TranslationZOffsetUnits=m  TranslationThetaOffset=0  TranslationThetaOffsetUnits=deg  RotationMethod=StandardAxis  RotationAngleUnits=rad  RotationStandardAxis=+Z  RotationAngle=Fi_b_z(6)  RotationArbitraryAxis=[0 0 1]  FollAlignAxisA=+X  BaseAlignAxisA=+Y  FollAlignAxisB=+Y  BaseAlignAxisB=+Z  RotationSequenceAxes=FollowerAxes  RotationSequence=XYX  RotationSequenceAngles=[0 0 0]  RotationSequenceAnglesUnits=deg  RotationMatrix=[1 0 0; 0 1 0; 0 0 1]
  trans z : sm_lib/Frames and Transforms/Rigid Transform  TranslationMethod=StandardAxis  TranslationStandardOffset=h_ub  TranslationLengthUnit=m  TranslationStandardAxis=-Z  TranslationCartesianOffset=[0 0 0]  TranslationROffset=0  TranslationROffsetUnits=m  TranslationZOffset=0  TranslationZOffsetUnits=m  TranslationThetaOffset=0  TranslationThetaOffsetUnits=deg  RotationMethod=None  RotationAngleUnits=deg  RotationStandardAxis=+Z  RotationAngle=0.0  RotationArbitraryAxis=[0 0 1]  FollAlignAxisA=+X  BaseAlignAxisA=+Y  FollAlignAxisB=+Y  BaseAlignAxisB=+Z  RotationSequenceAxes=FollowerAxes  RotationSequence=XYX  RotationSequenceAngles=[0 0 0]  RotationSequenceAnglesUnits=deg  RotationMatrix=[1 0 0; 0 1 0; 0 0 1]
  transl y : sm_lib/Frames and Transforms/Rigid Transform  TranslationMethod=StandardAxis  TranslationStandardOffset=w_ub/2  TranslationLengthUnit=m  TranslationStandardAxis=+Y  TranslationCartesianOffset=[0 0 0]  TranslationROffset=0  TranslationROffsetUnits=m  TranslationZOffset=0  TranslationZOffsetUnits=m  TranslationThetaOffset=0  TranslationThetaOffsetUnits=deg  RotationMethod=None  RotationAngleUnits=deg  RotationStandardAxis=+Z  RotationAngle=0.0  RotationArbitraryAxis=[0 0 1]  FollAlignAxisA=+X  BaseAlignAxisA=+Y  FollAlignAxisB=+Y  BaseAlignAxisB=+Z  RotationSequenceAxes=FollowerAxes  RotationSequence=XYX  RotationSequenceAngles=[0 0 0]  RotationSequenceAnglesUnits=deg  RotationMatrix=[1 0 0; 0 1 0; 0 0 1]
  O_ub : PMIOPort  Side=Left
  H_6 : PMIOPort  Port=2  Side=Right
  connections:
  trans z/LConn1 -- O_ub/RConn1
  trans z/RConn1 -- rot z/LConn1
  transl y/LConn1 -- rot z/RConn1
  transl y/RConn1 -- H_6/RConn1

== system iff_sim/High-authority control/CTC/computed torque control/bases + rods/lower base ==
  "O_lb -> G_1" : Subsystem
  "O_lb -> G_2" : Subsystem
  "O_lb -> G_3" : Subsystem
  body_lb : sm_lib/Body Elements/Extruded Solid  GraphicAmbientColor=[0.15 0.15 0.15 1.0]  BasedOnType=Density  CenterOfMass=[0 0 0]  CenterOfMassUnits=m  GraphicDiffuseColor=ctc_color  ExtrusionCrossSection=[1 1; -1 1; -1 -1; 1 -1]  ExtrusionCrossSectionUnits=m  Density=Ro_lb  DensityUnits=kg/m^3  DoExposeReferenceFrame=on  GraphicEmissiveColor=[0.0 0.0 0.0 1.0]  ExportEntireGeometry=off  ExtrusionLength=t_lb  ExtrusionLengthUnits=m  ExtrusionType=Regular  SerializedFrames=<Frames/>  MarkerShape=Sphere  MarkerSize=10  GraphicType=FromGeometry  InertiaType=CalculateFromGeometry  Mass=1  MassUnits=kg  MomentsOfInertia=[1 1 1]  MomentsOfInertiaUnits=kg*m^2  PolygonNumSides=6  GraphicOpacity=ctc_opacity  PolygonOuterRadius=(W_lb/2)/cosd(30)  PolygonOuterRadiusUnits=m  ProductsOfInertia=[0 0 0]  ProductsOfInertiaUnits=kg*m^2  GraphicShininess=75  GraphicSpecularColor=[0.5 0.5 0.5 1.0]  GraphicVisPropType=SimpleVisualProperties
      settings: SourceProductName=Simscape Multibody
  "wf -> O_lb" : Subsystem
  G_1 : PMIOPort  Side=Right
  G_2 : PMIOPort  Port=2  Side=Right
  G_3 : PMIOPort  Port=3  Side=Right
  wf : PMIOPort  Port=4  Side=Left
  connections:
  wf/RConn1 -- "wf -> O_lb"/LConn1
  "wf -> O_lb"/RConn1 -- "O_lb -> G_3"/LConn1 -- "O_lb -> G_2"/LConn1 -- body_lb/RConn1 -- "O_lb -> G_1"/LConn1
  G_1/RConn1 -- "O_lb -> G_1"/RConn1
  G_2/RConn1 -- "O_lb -> G_2"/RConn1
  "O_lb -> G_3"/RConn1 -- G_3/RConn1
